simulink model "VcScHv"  (R2023b)
settings: Solver=FixedStepDiscrete  StartTime=0.0  StopTime=1  FixedStep=0.01  RelTol=1e-3
model workspace (MAT data in the model file):
  K_VcScHv_BatteryVoltage_Fallback = Simulink.Parameter
  K_VcScHv_BatteryVoltage_Fallback.Value = 0
  K_VcScHv_BatteryVoltage_Fallback.Description = 'BatteryVoltage Fallback (V)'
  K_VcScHv_BatteryVoltage_Fallback.DataType = 'single'
  K_VcScHv_BatteryVoltage_Fallback.Min = 0
  K_VcScHv_BatteryVoltage_Fallback.Max = 1000
  K_VcScHv_BatteryVoltage_Fallback.Complexity = 'real'
  K_VcScHv_BatteryVoltage_Fallback.Dimensions = [1 1]
  K_VcScHv_BatteryVoltage_Maximum = Simulink.Parameter
  K_VcScHv_BatteryVoltage_Maximum.Value = 10000
  K_VcScHv_BatteryVoltage_Maximum.Description = 'BatteryVoltage Maximum (1)'
  K_VcScHv_BatteryVoltage_Maximum.DataType = 'uint16'
  K_VcScHv_BatteryVoltage_Maximum.Min = 0
  K_VcScHv_BatteryVoltage_Maximum.Max = 10000
  K_VcScHv_BatteryVoltage_Maximum.Complexity = 'real'
  K_VcScHv_BatteryVoltage_Maximum.Dimensions = [1 1]
  K_VcScHv_BatteryVoltage_Minimum = Simulink.Parameter
  K_VcScHv_BatteryVoltage_Minimum.Value = 0
  K_VcScHv_BatteryVoltage_Minimum.Description = 'BatteryVoltage Minimum (1)'
  K_VcScHv_BatteryVoltage_Minimum.DataType = 'uint16'
  K_VcScHv_BatteryVoltage_Minimum.Min = 0
  K_VcScHv_BatteryVoltage_Minimum.Max = 10000
  K_VcScHv_BatteryVoltage_Minimum.Complexity = 'real'
  K_VcScHv_BatteryVoltage_Minimum.Dimensions = [1 1]
  K_VcScHv_BatteryVoltage_Offset = Simulink.Parameter
  K_VcScHv_BatteryVoltage_Offset.Value = 0
  K_VcScHv_BatteryVoltage_Offset.Description = 'BatteryVoltage Offset (V)'
  K_VcScHv_BatteryVoltage_Offset.DataType = 'single'
  K_VcScHv_BatteryVoltage_Offset.Min = 0
  K_VcScHv_BatteryVoltage_Offset.Max = 1000
  K_VcScHv_BatteryVoltage_Offset.Complexity = 'real'
  K_VcScHv_BatteryVoltage_Offset.Dimensions = [1 1]
  K_VcScHv_BatteryVoltage_Scale = Simulink.Parameter
  K_VcScHv_BatteryVoltage_Scale.Value = 0.1
  K_VcScHv_BatteryVoltage_Scale.Description = 'BatteryVoltage Scale (1)'
  K_VcScHv_BatteryVoltage_Scale.DataType = 'single'
  K_VcScHv_BatteryVoltage_Scale.Min = 0
  K_VcScHv_BatteryVoltage_Scale.Max = 100
  K_VcScHv_BatteryVoltage_Scale.Complexity = 'real'
  K_VcScHv_BatteryVoltage_Scale.Dimensions = [1 1]
  K_VcScHv_BatteryVoltage_Timeout = Simulink.Parameter
  K_VcScHv_BatteryVoltage_Timeout.Value = 0.05
  K_VcScHv_BatteryVoltage_Timeout.Description = 'BatteryVoltage Timeout (s)'
  K_VcScHv_BatteryVoltage_Timeout.DataType = 'single'
  K_VcScHv_BatteryVoltage_Timeout.Min = 0
  K_VcScHv_BatteryVoltage_Timeout.Max = 10
  K_VcScHv_BatteryVoltage_Timeout.Complexity = 'real'
  K_VcScHv_BatteryVoltage_Timeout.Dimensions = [1 1]
  K_VcScHv_ChargeEnable_Fallback = Simulink.Parameter
  K_VcScHv_ChargeEnable_Fallback.Value = 0
  K_VcScHv_ChargeEnable_Fallback.Description = 'ChargeEnable Fallback (boolean)'
  K_VcScHv_ChargeEnable_Fallback.DataType = 'boolean'
  K_VcScHv_ChargeEnable_Fallback.Min = 0
  K_VcScHv_ChargeEnable_Fallback.Max = 1
  K_VcScHv_ChargeEnable_Fallback.Complexity = 'real'
  K_VcScHv_ChargeEnable_Fallback.Dimensions = [1 1]
  K_VcScHv_ChargeEnable_Timeout = Simulink.Parameter
  K_VcScHv_ChargeEnable_Timeout.Value = 0.05
  K_VcScHv_ChargeEnable_Timeout.Description = 'ChargeEnable Timeout (s)'
  K_VcScHv_ChargeEnable_Timeout.DataType = 'single'
  K_VcScHv_ChargeEnable_Timeout.Min = 0
  K_VcScHv_ChargeEnable_Timeout.Max = 10
  K_VcScHv_ChargeEnable_Timeout.Complexity = 'real'
  K_VcScHv_ChargeEnable_Timeout.Dimensions = [1 1]
  K_VcScHv_ContactorFeedback_Fallback = Simulink.Parameter
  K_VcScHv_ContactorFeedback_Fallback.Value = 0
  K_VcScHv_ContactorFeedback_Fallback.Description = 'ContactorFeedback Fallback (boolean)'
  K_VcScHv_ContactorFeedback_Fallback.DataType = 'boolean'
  K_VcScHv_ContactorFeedback_Fallback.Min = 0
  K_VcScHv_ContactorFeedback_Fallback.Max = 1
  K_VcScHv_ContactorFeedback_Fallback.Complexity = 'real'
  K_VcScHv_ContactorFeedback_Fallback.Dimensions = [1 1]
  K_VcScHv_ContactorFeedback_Timeout = Simulink.Parameter
  K_VcScHv_ContactorFeedback_Timeout.Value = 0.05
  K_VcScHv_ContactorFeedback_Timeout.Description = 'ContactorFeedback Timeout (s)'
  K_VcScHv_ContactorFeedback_Timeout.DataType = 'single'
  K_VcScHv_ContactorFeedback_Timeout.Min = 0
  K_VcScHv_ContactorFeedback_Timeout.Max = 10
  K_VcScHv_ContactorFeedback_Timeout.Complexity = 'real'
  K_VcScHv_ContactorFeedback_Timeout.Dimensions = [1 1]
  K_VcScHv_CrashSignal_Fallback = Simulink.Parameter
  K_VcScHv_CrashSignal_Fallback.Value = 1
  K_VcScHv_CrashSignal_Fallback.Description = 'CrashSignal Fallback (boolean)'
  K_VcScHv_CrashSignal_Fallback.DataType = 'boolean'
  K_VcScHv_CrashSignal_Fallback.Min = 0
  K_VcScHv_CrashSignal_Fallback.Max = 1
  K_VcScHv_CrashSignal_Fallback.Complexity = 'real'
  K_VcScHv_CrashSignal_Fallback.Dimensions = [1 1]
  K_VcScHv_CrashSignal_Timeout = Simulink.Parameter
  K_VcScHv_CrashSignal_Timeout.Value = 0.05
  K_VcScHv_CrashSignal_Timeout.Description = 'CrashSignal Timeout (s)'
  K_VcScHv_CrashSignal_Timeout.DataType = 'single'
  K_VcScHv_CrashSignal_Timeout.Min = 0
  K_VcScHv_CrashSignal_Timeout.Max = 10
  K_VcScHv_CrashSignal_Timeout.Complexity = 'real'
  K_VcScHv_CrashSignal_Timeout.Dimensions = [1 1]
  K_VcScHv_DcLinkVoltage_Fallback = Simulink.Parameter
  K_VcScHv_DcLinkVoltage_Fallback.Value = 0
  K_VcScHv_DcLinkVoltage_Fallback.Description = 'DcLinkVoltage Fallback (V)'
  K_VcScHv_DcLinkVoltage_Fallback.DataType = 'single'
  K_VcScHv_DcLinkVoltage_Fallback.Min = 0
  K_VcScHv_DcLinkVoltage_Fallback.Max = 1000
  K_VcScHv_DcLinkVoltage_Fallback.Complexity = 'real'
  K_VcScHv_DcLinkVoltage_Fallback.Dimensions = [1 1]
  K_VcScHv_DcLinkVoltage_Maximum = Simulink.Parameter
  K_VcScHv_DcLinkVoltage_Maximum.Value = 10000
  K_VcScHv_DcLinkVoltage_Maximum.Description = 'DcLinkVoltage Maximum (1)'
  K_VcScHv_DcLinkVoltage_Maximum.DataType = 'uint16'
  K_VcScHv_DcLinkVoltage_Maximum.Min = 0
  K_VcScHv_DcLinkVoltage_Maximum.Max = 10000
  K_VcScHv_DcLinkVoltage_Maximum.Complexity = 'real'
  K_VcScHv_DcLinkVoltage_Maximum.Dimensions = [1 1]
  K_VcScHv_DcLinkVoltage_Minimum = Simulink.Parameter
  K_VcScHv_DcLinkVoltage_Minimum.Value = 0
  K_VcScHv_DcLinkVoltage_Minimum.Description = 'DcLinkVoltage Minimum (1)'
  K_VcScHv_DcLinkVoltage_Minimum.DataType = 'uint16'
  K_VcScHv_DcLinkVoltage_Minimum.Min = 0
  K_VcScHv_DcLinkVoltage_Minimum.Max = 10000
  K_VcScHv_DcLinkVoltage_Minimum.Complexity = 'real'
  K_VcScHv_DcLinkVoltage_Minimum.Dimensions = [1 1]
  K_VcScHv_DcLinkVoltage_Offset = Simulink.Parameter
  K_VcScHv_DcLinkVoltage_Offset.Value = 0
  K_VcScHv_DcLinkVoltage_Offset.Description = 'DcLinkVoltage Offset (V)'
  K_VcScHv_DcLinkVoltage_Offset.DataType = 'single'
  K_VcScHv_DcLinkVoltage_Offset.Min = 0
  K_VcScHv_DcLinkVoltage_Offset.Max = 1000
  K_VcScHv_DcLinkVoltage_Offset.Complexity = 'real'
  K_VcScHv_DcLinkVoltage_Offset.Dimensions = [1 1]
  K_VcScHv_DcLinkVoltage_Scale = Simulink.Parameter
  K_VcScHv_DcLinkVoltage_Scale.Value = 0.1
  K_VcScHv_DcLinkVoltage_Scale.Description = 'DcLinkVoltage Scale (1)'
  K_VcScHv_DcLinkVoltage_Scale.DataType = 'single'
  K_VcScHv_DcLinkVoltage_Scale.Min = 0
  K_VcScHv_DcLinkVoltage_Scale.Max = 100
  K_VcScHv_DcLinkVoltage_Scale.Complexity = 'real'
  K_VcScHv_DcLinkVoltage_Scale.Dimensions = [1 1]
  K_VcScHv_DcLinkVoltage_Timeout = Simulink.Parameter
  K_VcScHv_DcLinkVoltage_Timeout.Value = 0.05
  K_VcScHv_DcLinkVoltage_Timeout.Description = 'DcLinkVoltage Timeout (s)'
  K_VcScHv_DcLinkVoltage_Timeout.DataType = 'single'
  K_VcScHv_DcLinkVoltage_Timeout.Min = 0
  K_VcScHv_DcLinkVoltage_Timeout.Max = 10
  K_VcScHv_DcLinkVoltage_Timeout.Complexity = 'real'
  K_VcScHv_DcLinkVoltage_Timeout.Dimensions = [1 1]
  K_VcScHv_DriveEnable_Fallback = Simulink.Parameter
  K_VcScHv_DriveEnable_Fallback.Value = 0
  K_VcScHv_DriveEnable_Fallback.Description = 'DriveEnable Fallback (boolean)'
  K_VcScHv_DriveEnable_Fallback.DataType = 'boolean'
  K_VcScHv_DriveEnable_Fallback.Min = 0
  K_VcScHv_DriveEnable_Fallback.Max = 1
  K_VcScHv_DriveEnable_Fallback.Complexity = 'real'
  K_VcScHv_DriveEnable_Fallback.Dimensions = [1 1]
  K_VcScHv_DriveEnable_Timeout = Simulink.Parameter
  K_VcScHv_DriveEnable_Timeout.Value = 0.05
  K_VcScHv_DriveEnable_Timeout.Description = 'DriveEnable Timeout (s)'
  K_VcScHv_DriveEnable_Timeout.DataType = 'single'
  K_VcScHv_DriveEnable_Timeout.Min = 0
  K_VcScHv_DriveEnable_Timeout.Max = 10
  K_VcScHv_DriveEnable_Timeout.Complexity = 'real'
  K_VcScHv_DriveEnable_Timeout.Dimensions = [1 1]
  K_VcScHv_IsolationResistance_Fallback = Simulink.Parameter
  K_VcScHv_IsolationResistance_Fallback.Value = 0
  K_VcScHv_IsolationResistance_Fallback.Description = 'IsolationResistance Fallback (ohm)'
  K_VcScHv_IsolationResistance_Fallback.DataType = 'single'
  K_VcScHv_IsolationResistance_Fallback.Min = 0
  K_VcScHv_IsolationResistance_Fallback.Max = 2000000
  K_VcScHv_IsolationResistance_Fallback.Complexity = 'real'
  K_VcScHv_IsolationResistance_Fallback.Dimensions = [1 1]
  K_VcScHv_IsolationResistance_Maximum = Simulink.Parameter
  K_VcScHv_IsolationResistance_Maximum.Value = 2000000
  K_VcScHv_IsolationResistance_Maximum.Description = 'IsolationResistance Maximum (ohm)'
  K_VcScHv_IsolationResistance_Maximum.DataType = 'uint32'
  K_VcScHv_IsolationResistance_Maximum.Min = 0
  K_VcScHv_IsolationResistance_Maximum.Max = 2000000
  K_VcScHv_IsolationResistance_Maximum.Complexity = 'real'
  K_VcScHv_IsolationResistance_Maximum.Dimensions = [1 1]
  K_VcScHv_IsolationResistance_Minimum = Simulink.Parameter
  K_VcScHv_IsolationResistance_Minimum.Value = 0
  K_VcScHv_IsolationResistance_Minimum.Description = 'IsolationResistance Minimum (ohm)'
  K_VcScHv_IsolationResistance_Minimum.DataType = 'uint32'
  K_VcScHv_IsolationResistance_Minimum.Min = 0
  K_VcScHv_IsolationResistance_Minimum.Max = 2000000
  K_VcScHv_IsolationResistance_Minimum.Complexity = 'real'
  K_VcScHv_IsolationResistance_Minimum.Dimensions = [1 1]
  K_VcScHv_IsolationResistance_Offset = Simulink.Parameter
  K_VcScHv_IsolationResistance_Offset.Value = 0
  K_VcScHv_IsolationResistance_Offset.Description = 'IsolationResistance Offset (ohm)'
  K_VcScHv_IsolationResistance_Offset.DataType = 'single'
  K_VcScHv_IsolationResistance_Offset.Min = 0
  K_VcScHv_IsolationResistance_Offset.Max = 2000000
  K_VcScHv_IsolationResistance_Offset.Complexity = 'real'
  K_VcScHv_IsolationResistance_Offset.Dimensions = [1 1]
  K_VcScHv_IsolationResistance_Scale = Simulink.Parameter
  K_VcScHv_IsolationResistance_Scale.Value = 1
  K_VcScHv_IsolationResistance_Scale.Description = 'IsolationResistance Scale (1)'
  K_VcScHv_IsolationResistance_Scale.DataType = 'single'
  K_VcScHv_IsolationResistance_Scale.Min = 0
  K_VcScHv_IsolationResistance_Scale.Max = 100
  K_VcScHv_IsolationResistance_Scale.Complexity = 'real'
  K_VcScHv_IsolationResistance_Scale.Dimensions = [1 1]
  K_VcScHv_IsolationResistance_Timeout = Simulink.Parameter
  K_VcScHv_IsolationResistance_Timeout.Value = 0.05
  K_VcScHv_IsolationResistance_Timeout.Description = 'IsolationResistance Timeout (s)'
  K_VcScHv_IsolationResistance_Timeout.DataType = 'single'
  K_VcScHv_IsolationResistance_Timeout.Min = 0
  K_VcScHv_IsolationResistance_Timeout.Max = 10
  K_VcScHv_IsolationResistance_Timeout.Complexity = 'real'
  K_VcScHv_IsolationResistance_Timeout.Dimensions = [1 1]
  K_VcScHv_PrechargeFeedback_Fallback = Simulink.Parameter
  K_VcScHv_PrechargeFeedback_Fallback.Value = 0
  K_VcScHv_PrechargeFeedback_Fallback.Description = 'PrechargeFeedback Fallback (boolean)'
  K_VcScHv_PrechargeFeedback_Fallback.DataType = 'boolean'
  K_VcScHv_PrechargeFeedback_Fallback.Min = 0
  K_VcScHv_PrechargeFeedback_Fallback.Max = 1
  K_VcScHv_PrechargeFeedback_Fallback.Complexity = 'real'
  K_VcScHv_PrechargeFeedback_Fallback.Dimensions = [1 1]
  K_VcScHv_PrechargeFeedback_Timeout = Simulink.Parameter
  K_VcScHv_PrechargeFeedback_Timeout.Value = 0.05
  K_VcScHv_PrechargeFeedback_Timeout.Description = 'PrechargeFeedback Timeout (s)'
  K_VcScHv_PrechargeFeedback_Timeout.DataType = 'single'
  K_VcScHv_PrechargeFeedback_Timeout.Min = 0
  K_VcScHv_PrechargeFeedback_Timeout.Max = 10
  K_VcScHv_PrechargeFeedback_Timeout.Complexity = 'real'
  K_VcScHv_PrechargeFeedback_Timeout.Dimensions = [1 1]
libraries: simulink x1
(part 1 of 2)
Description:
  | Synthetic reality proxy: high_voltage_sequence. Local engineering values; not internal production calibration.
settings Model: Creator=曹博弢  LastModifiedBy=曹博弢
settings DataIOCC: SignalLogging=off
settings OptimizationCC: EnhancedBackFolding=on  PassReuseOutputArgsAs=Individual arguments  ZeroExternalMemoryAtStartup=off  ZeroInternalMemoryAtStartup=off  OptimizeBlockOrder=speed  DifferentSizesBufferReuse=on  OptimizationCustomize=off  EfficientTunableParamExpr=on
settings DebuggingCC: ParameterTunabilityLossMsg=error
settings SFSimCC: MATLABDynamicMemAlloc=off
settings RTWCC: Description=Embedded Coder  SystemTargetFile=ert.tlc  GenCodeOnly=on  TemplateMakefile=ert_default_tmf
settings CodeAppCC: ForceParamTrailComments=on  IgnoreCustomStorageClasses=off  OperatorAnnotations=on  SimulinkDataObjDesc=on  SFDataObjDesc=on  InsertBlockDesc=on
settings ERTTargetCC: TargetLangStandard=C99 (ISO)  GenerateSampleERTMain=on  ERTCustomFileTemplate=example_file_process.tlc

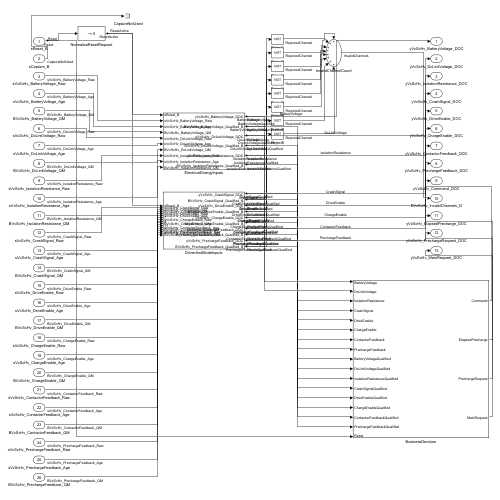
[thumbnail: Simulink's stored preview of the top-level diagram]
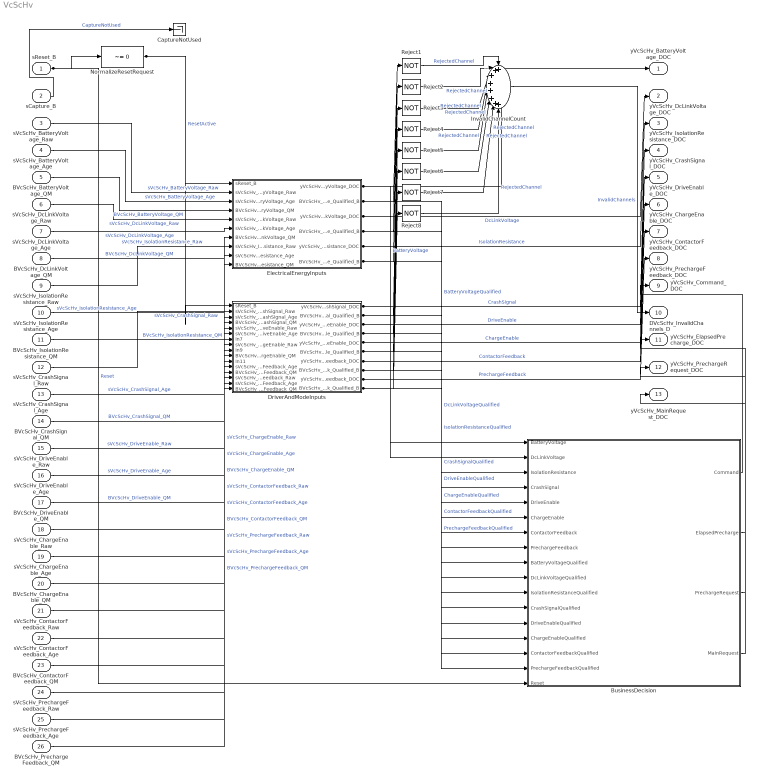
== system VcScHv ==
  sReset_B : Inport  OutDataTypeStr=boolean  Interpolate=off
  sCapture_B : Inport  Port=2  OutDataTypeStr=boolean  Interpolate=off
  sVcScHv_BatteryVoltage_Raw : Inport  Port=3  OutDataTypeStr=uint16  Interpolate=off
  sVcScHv_BatteryVoltage_Age : Inport  Port=4  OutDataTypeStr=single  Interpolate=off
  BVcScHv_BatteryVoltage_QM : Inport  Port=5  OutDataTypeStr=boolean  Interpolate=off
  sVcScHv_DcLinkVoltage_Raw : Inport  Port=6  OutDataTypeStr=uint16  Interpolate=off
  sVcScHv_DcLinkVoltage_Age : Inport  Port=7  OutDataTypeStr=single  Interpolate=off
  BVcScHv_DcLinkVoltage_QM : Inport  Port=8  OutDataTypeStr=boolean  Interpolate=off
  sVcScHv_IsolationResistance_Raw : Inport  Port=9  OutDataTypeStr=uint32  Interpolate=off
  sVcScHv_IsolationResistance_Age : Inport  Port=10  OutDataTypeStr=single  Interpolate=off
  BVcScHv_IsolationResistance_QM : Inport  Port=11  OutDataTypeStr=boolean  Interpolate=off
  sVcScHv_CrashSignal_Raw : Inport  Port=12  OutDataTypeStr=boolean  Interpolate=off
  sVcScHv_CrashSignal_Age : Inport  Port=13  OutDataTypeStr=single  Interpolate=off
  BVcScHv_CrashSignal_QM : Inport  Port=14  OutDataTypeStr=boolean  Interpolate=off
  sVcScHv_DriveEnable_Raw : Inport  Port=15  OutDataTypeStr=boolean  Interpolate=off
  sVcScHv_DriveEnable_Age : Inport  Port=16  OutDataTypeStr=single  Interpolate=off
  BVcScHv_DriveEnable_QM : Inport  Port=17  OutDataTypeStr=boolean  Interpolate=off
  sVcScHv_ChargeEnable_Raw : Inport  Port=18  OutDataTypeStr=boolean  Interpolate=off
  sVcScHv_ChargeEnable_Age : Inport  Port=19  OutDataTypeStr=single  Interpolate=off
  BVcScHv_ChargeEnable_QM : Inport  Port=20  OutDataTypeStr=boolean  Interpolate=off
  sVcScHv_ContactorFeedback_Raw : Inport  Port=21  OutDataTypeStr=boolean  Interpolate=off
  sVcScHv_ContactorFeedback_Age : Inport  Port=22  OutDataTypeStr=single  Interpolate=off
  BVcScHv_ContactorFeedback_QM : Inport  Port=23  OutDataTypeStr=boolean  Interpolate=off
  sVcScHv_PrechargeFeedback_Raw : Inport  Port=24  OutDataTypeStr=boolean  Interpolate=off
  sVcScHv_PrechargeFeedback_Age : Inport  Port=25  OutDataTypeStr=single  Interpolate=off
  BVcScHv_PrechargeFeedback_QM : Inport  Port=26  OutDataTypeStr=boolean  Interpolate=off
  BusinessDecision : Subsystem
  CaptureNotUsed : Terminator
  DriverAndModeInputs : Subsystem
  ElectricalEnergyInputs : Subsystem
  InvalidChannelCount : Sum  Inputs=++++++++  OutDataTypeStr=uint16
  NormalizeResetRequest : simulink/Logic and Bit Operations/Compare To Zero  relop=~=  OutDataTypeStr=boolean
  Reject{1..8} (8 alike) : Logic  Operator=NOT  AllPortsSameDT=off  OutDataTypeStr=boolean
  yVcScHv_BatteryVoltage_DOC : Outport
  yVcScHv_DcLinkVoltage_DOC : Outport  Port=2
  yVcScHv_IsolationResistance_DOC : Outport  Port=3
  yVcScHv_CrashSignal_DOC : Outport  Port=4
  yVcScHv_DriveEnable_DOC : Outport  Port=5
  yVcScHv_ChargeEnable_DOC : Outport  Port=6
  yVcScHv_ContactorFeedback_DOC : Outport  Port=7
  yVcScHv_PrechargeFeedback_DOC : Outport  Port=8
  yVcScHv_Command_DOC : Outport  Port=9
  DVcScHv_InvalidChannels_D : Outport  Port=10
  yVcScHv_ElapsedPrecharge_DOC : Outport  Port=11
  yVcScHv_PrechargeRequest_DOC : Outport  Port=12
  yVcScHv_MainRequest_DOC : Outport  Port=13
  wires:
  sVcScHv_BatteryVoltage_Raw/1 -> ElectricalEnergyInputs/2(sVcScHv_BatteryVoltage_Raw)  "sVcScHv_BatteryVoltage_Raw"
  sVcScHv_BatteryVoltage_Age/1 -> ElectricalEnergyInputs/3(sVcScHv_BatteryVoltage_Age)  "sVcScHv_BatteryVoltage_Age"
  BVcScHv_BatteryVoltage_QM/1 -> ElectricalEnergyInputs/4(BVcScHv_BatteryVoltage_QM)  "BVcScHv_BatteryVoltage_QM"
  sVcScHv_DcLinkVoltage_Raw/1 -> ElectricalEnergyInputs/5(sVcScHv_DcLinkVoltage_Raw)  "sVcScHv_DcLinkVoltage_Raw"
  sVcScHv_DcLinkVoltage_Age/1 -> ElectricalEnergyInputs/6(sVcScHv_DcLinkVoltage_Age)  "sVcScHv_DcLinkVoltage_Age"
  BVcScHv_DcLinkVoltage_QM/1 -> ElectricalEnergyInputs/7(BVcScHv_DcLinkVoltage_QM)  "BVcScHv_DcLinkVoltage_QM"
  sVcScHv_IsolationResistance_Raw/1 -> ElectricalEnergyInputs/8(sVcScHv_IsolationResistance_Raw)  "sVcScHv_IsolationResistance_Raw"
  sVcScHv_IsolationResistance_Age/1 -> ElectricalEnergyInputs/9(sVcScHv_IsolationResistance_Age)  "sVcScHv_IsolationResistance_Age"
  BVcScHv_IsolationResistance_QM/1 -> ElectricalEnergyInputs/10(BVcScHv_IsolationResistance_QM)  "BVcScHv_IsolationResistance_QM"
  sVcScHv_CrashSignal_Raw/1 -> DriverAndModeInputs/2(sVcScHv_CrashSignal_Raw)  "sVcScHv_CrashSignal_Raw"
  sVcScHv_CrashSignal_Age/1 -> DriverAndModeInputs/3(sVcScHv_CrashSignal_Age)  "sVcScHv_CrashSignal_Age"
  BVcScHv_CrashSignal_QM/1 -> DriverAndModeInputs/4(BVcScHv_CrashSignal_QM)  "BVcScHv_CrashSignal_QM"
  sVcScHv_DriveEnable_Raw/1 -> DriverAndModeInputs/5(sVcScHv_DriveEnable_Raw)  "sVcScHv_DriveEnable_Raw"
  sVcScHv_DriveEnable_Age/1 -> DriverAndModeInputs/6(sVcScHv_DriveEnable_Age)  "sVcScHv_DriveEnable_Age"
  BVcScHv_DriveEnable_QM/1 -> DriverAndModeInputs/7(In7)  "BVcScHv_DriveEnable_QM"
  sVcScHv_ChargeEnable_Raw/1 -> DriverAndModeInputs/8(sVcScHv_ChargeEnable_Raw)  "sVcScHv_ChargeEnable_Raw"
  sVcScHv_ChargeEnable_Age/1 -> DriverAndModeInputs/9(In9)  "sVcScHv_ChargeEnable_Age"
  BVcScHv_ChargeEnable_QM/1 -> DriverAndModeInputs/10(BVcScHv_ChargeEnable_QM)  "BVcScHv_ChargeEnable_QM"
  sVcScHv_ContactorFeedback_Raw/1 -> DriverAndModeInputs/11(In11)  "sVcScHv_ContactorFeedback_Raw"
  sVcScHv_ContactorFeedback_Age/1 -> DriverAndModeInputs/12(sVcScHv_ContactorFeedback_Age)  "sVcScHv_ContactorFeedback_Age"
  BVcScHv_ContactorFeedback_QM/1 -> DriverAndModeInputs/13(BVcScHv_ContactorFeedback_QM)  "BVcScHv_ContactorFeedback_QM"
  sVcScHv_PrechargeFeedback_Raw/1 -> DriverAndModeInputs/14(sVcScHv_PrechargeFeedback_Raw)  "sVcScHv_PrechargeFeedback_Raw"
  sVcScHv_PrechargeFeedback_Age/1 -> DriverAndModeInputs/15(sVcScHv_PrechargeFeedback_Age)  "sVcScHv_PrechargeFeedback_Age"
  BVcScHv_PrechargeFeedback_QM/1 -> DriverAndModeInputs/16(BVcScHv_PrechargeFeedback_QM)  "BVcScHv_PrechargeFeedback_QM"
  ElectricalEnergyInputs/1(yVcScHv_BatteryVoltage_DOC) -> yVcScHv_BatteryVoltage_DOC/1, BusinessDecision/1(BatteryVoltage)  "BatteryVoltage"
  ElectricalEnergyInputs/3(yVcScHv_DcLinkVoltage_DOC) -> yVcScHv_DcLinkVoltage_DOC/1, BusinessDecision/2(DcLinkVoltage)  "DcLinkVoltage"
  ElectricalEnergyInputs/5(yVcScHv_IsolationResistance_DOC) -> yVcScHv_IsolationResistance_DOC/1, BusinessDecision/3(IsolationResistance)  "IsolationResistance"
  DriverAndModeInputs/1(yVcScHv_CrashSignal_DOC) -> yVcScHv_CrashSignal_DOC/1, BusinessDecision/4(CrashSignal)  "CrashSignal"
  DriverAndModeInputs/3(yVcScHv_DriveEnable_DOC) -> yVcScHv_DriveEnable_DOC/1, BusinessDecision/5(DriveEnable)  "DriveEnable"
  DriverAndModeInputs/5(yVcScHv_ChargeEnable_DOC) -> yVcScHv_ChargeEnable_DOC/1, BusinessDecision/6(ChargeEnable)  "ChargeEnable"
  DriverAndModeInputs/7(yVcScHv_ContactorFeedback_DOC) -> yVcScHv_ContactorFeedback_DOC/1, BusinessDecision/7(ContactorFeedback)  "ContactorFeedback"
  DriverAndModeInputs/9(yVcScHv_PrechargeFeedback_DOC) -> yVcScHv_PrechargeFeedback_DOC/1, BusinessDecision/8(PrechargeFeedback)  "PrechargeFeedback"
  ElectricalEnergyInputs/2(BVcScHv_BatteryVoltage_Qualified_B) -> Reject1/1, BusinessDecision/9(BatteryVoltageQualified)  "BatteryVoltageQualified"
  Reject1/1 -> InvalidChannelCount/1  "RejectedChannel"
  ElectricalEnergyInputs/4(BVcScHv_DcLinkVoltage_Qualified_B) -> Reject2/1, BusinessDecision/10(DcLinkVoltageQualified)  "DcLinkVoltageQualified"
  Reject2/1 -> InvalidChannelCount/2  "RejectedChannel"
  ElectricalEnergyInputs/6(BVcScHv_IsolationResistance_Qualified_B) -> Reject3/1, BusinessDecision/11(IsolationResistanceQualified)  "IsolationResistanceQualified"
  Reject3/1 -> InvalidChannelCount/3  "RejectedChannel"
  DriverAndModeInputs/2(BVcScHv_CrashSignal_Qualified_B) -> Reject4/1, BusinessDecision/12(CrashSignalQualified)  "CrashSignalQualified"
  Reject4/1 -> InvalidChannelCount/4  "RejectedChannel"
  DriverAndModeInputs/4(BVcScHv_DriveEnable_Qualified_B) -> Reject5/1, BusinessDecision/13(DriveEnableQualified)  "DriveEnableQualified"
  Reject5/1 -> InvalidChannelCount/5  "RejectedChannel"
  DriverAndModeInputs/6(BVcScHv_ChargeEnable_Qualified_B) -> Reject6/1, BusinessDecision/14(ChargeEnableQualified)  "ChargeEnableQualified"
  Reject6/1 -> InvalidChannelCount/6  "RejectedChannel"
  DriverAndModeInputs/8(BVcScHv_ContactorFeedback_Qualified_B) -> Reject7/1, BusinessDecision/15(ContactorFeedbackQualified)  "ContactorFeedbackQualified"
  Reject7/1 -> InvalidChannelCount/7  "RejectedChannel"
  DriverAndModeInputs/10(BVcScHv_PrechargeFeedback_Qualified_B) -> Reject8/1, BusinessDecision/16(PrechargeFeedbackQualified)  "PrechargeFeedbackQualified"
  Reject8/1 -> InvalidChannelCount/8  "RejectedChannel"
  InvalidChannelCount/1 -> DVcScHv_InvalidChannels_D/1  "InvalidChannels"
  sCapture_B/1 -> CaptureNotUsed/1  "CaptureNotUsed"
  sReset_B/1 -> NormalizeResetRequest/1, BusinessDecision/17(Reset)  "Reset"
  NormalizeResetRequest/1 -> ElectricalEnergyInputs/1(sReset_B), DriverAndModeInputs/1(sReset_B)  "ResetActive"
  BusinessDecision/1(Command) -> yVcScHv_Command_DOC/1
  BusinessDecision/2(ElapsedPrecharge) -> yVcScHv_ElapsedPrecharge_DOC/1
  BusinessDecision/3(PrechargeRequest) -> yVcScHv_PrechargeRequest_DOC/1
  BusinessDecision/4(MainRequest) -> yVcScHv_MainRequest_DOC/1

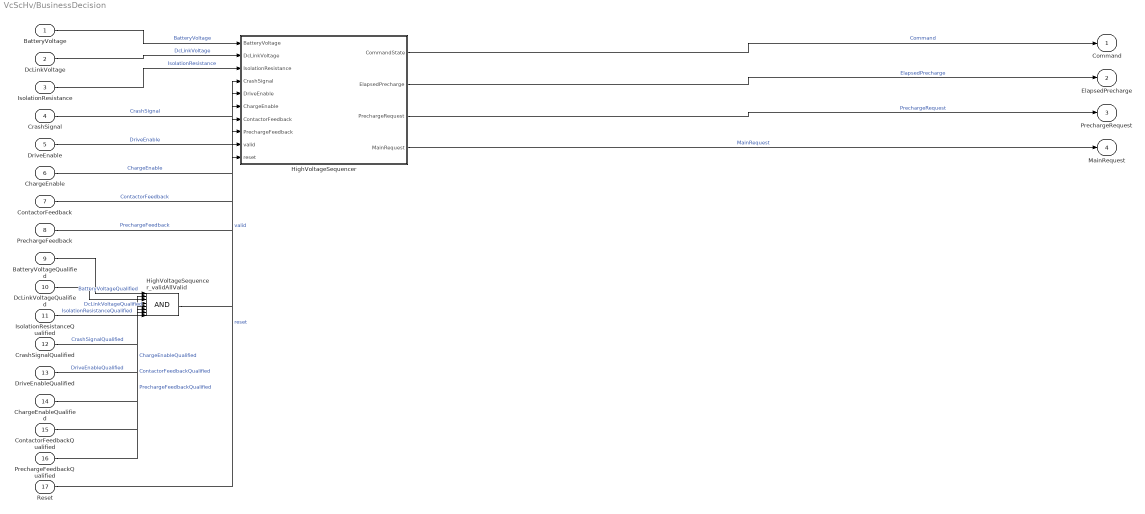
== system VcScHv/BusinessDecision ==
  BatteryVoltage : Inport
  DcLinkVoltage : Inport  Port=2
  IsolationResistance : Inport  Port=3
  CrashSignal : Inport  Port=4
  DriveEnable : Inport  Port=5
  ChargeEnable : Inport  Port=6
  ContactorFeedback : Inport  Port=7
  PrechargeFeedback : Inport  Port=8
  BatteryVoltageQualified : Inport  Port=9
  DcLinkVoltageQualified : Inport  Port=10
  IsolationResistanceQualified : Inport  Port=11
  CrashSignalQualified : Inport  Port=12
  DriveEnableQualified : Inport  Port=13
  ChargeEnableQualified : Inport  Port=14
  ContactorFeedbackQualified : Inport  Port=15
  PrechargeFeedbackQualified : Inport  Port=16
  Reset : Inport  Port=17
  HighVoltageSequencer : Subsystem  Description=Executable responsibility: HighVoltageSequencer. Port units and scenarios are in BusinessBehavior.md and the interface workbook.
  HighVoltageSequencer_validAllValid : Logic  Inputs=8  AllPortsSameDT=off  OutDataTypeStr=boolean
  Command : Outport
  ElapsedPrecharge : Outport  Port=2
  PrechargeRequest : Outport  Port=3
  MainRequest : Outport  Port=4
  wires:
  BatteryVoltage/1 -> HighVoltageSequencer/1(BatteryVoltage)  "BatteryVoltage"
  DcLinkVoltage/1 -> HighVoltageSequencer/2(DcLinkVoltage)  "DcLinkVoltage"
  IsolationResistance/1 -> HighVoltageSequencer/3(IsolationResistance)  "IsolationResistance"
  CrashSignal/1 -> HighVoltageSequencer/4(CrashSignal)  "CrashSignal"
  DriveEnable/1 -> HighVoltageSequencer/5(DriveEnable)  "DriveEnable"
  ChargeEnable/1 -> HighVoltageSequencer/6(ChargeEnable)  "ChargeEnable"
  ContactorFeedback/1 -> HighVoltageSequencer/7(ContactorFeedback)  "ContactorFeedback"
  PrechargeFeedback/1 -> HighVoltageSequencer/8(PrechargeFeedback)  "PrechargeFeedback"
  BatteryVoltageQualified/1 -> HighVoltageSequencer_validAllValid/1  "BatteryVoltageQualified"
  DcLinkVoltageQualified/1 -> HighVoltageSequencer_validAllValid/2  "DcLinkVoltageQualified"
  IsolationResistanceQualified/1 -> HighVoltageSequencer_validAllValid/3  "IsolationResistanceQualified"
  CrashSignalQualified/1 -> HighVoltageSequencer_validAllValid/4  "CrashSignalQualified"
  DriveEnableQualified/1 -> HighVoltageSequencer_validAllValid/5  "DriveEnableQualified"
  ChargeEnableQualified/1 -> HighVoltageSequencer_validAllValid/6  "ChargeEnableQualified"
  ContactorFeedbackQualified/1 -> HighVoltageSequencer_validAllValid/7  "ContactorFeedbackQualified"
  PrechargeFeedbackQualified/1 -> HighVoltageSequencer_validAllValid/8  "PrechargeFeedbackQualified"
  HighVoltageSequencer_validAllValid/1 -> HighVoltageSequencer/9(valid)  "valid"
  Reset/1 -> HighVoltageSequencer/10(reset)  "reset"
  HighVoltageSequencer/1(CommandState) -> Command/1  "Command"
  HighVoltageSequencer/2(ElapsedPrecharge) -> ElapsedPrecharge/1  "ElapsedPrecharge"
  HighVoltageSequencer/3(PrechargeRequest) -> PrechargeRequest/1  "PrechargeRequest"
  HighVoltageSequencer/4(MainRequest) -> MainRequest/1  "MainRequest"

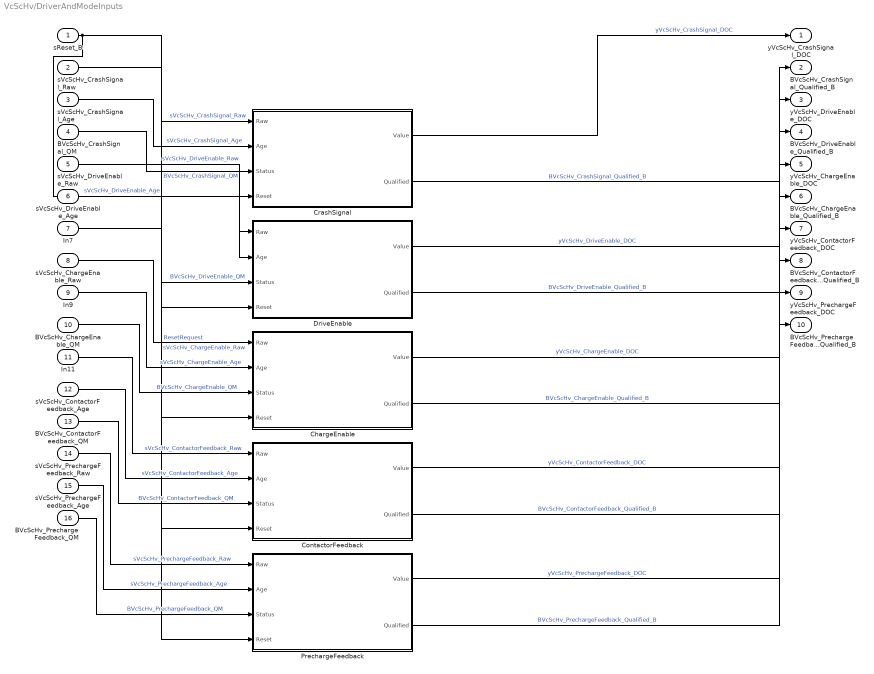
== system VcScHv/DriverAndModeInputs ==
  sReset_B : Inport
  sVcScHv_CrashSignal_Raw : Inport  Port=2
  sVcScHv_CrashSignal_Age : Inport  Port=3
  BVcScHv_CrashSignal_QM : Inport  Port=4
  sVcScHv_DriveEnable_Raw : Inport  Port=5
  sVcScHv_DriveEnable_Age : Inport  Port=6
  In7 : Inport  Port=7
  sVcScHv_ChargeEnable_Raw : Inport  Port=8
  In9 : Inport  Port=9
  BVcScHv_ChargeEnable_QM : Inport  Port=10
  In11 : Inport  Port=11
  sVcScHv_ContactorFeedback_Age : Inport  Port=12
  BVcScHv_ContactorFeedback_QM : Inport  Port=13
  sVcScHv_PrechargeFeedback_Raw : Inport  Port=14
  sVcScHv_PrechargeFeedback_Age : Inport  Port=15
  BVcScHv_PrechargeFeedback_QM : Inport  Port=16
  ChargeEnable : Subsystem  Description=ChargeEnable: digital qualification; raw=boolean, physical=boolean, physical=raw*1+0 boolean  mask{ChannelTimeout=K_VcScHv_ChargeEnable_Timeout}
      mask prompts: ChannelTimeout "Timeout"
      mask help: ChargeEnable: digital qualification; raw=boolean, physical=boolean, physical=raw*1+0 boolean
  ContactorFeedback : Subsystem  Description=ContactorFeedback: digital qualification; raw=boolean, physical=boolean, physical=raw*1+0 boolean  mask{ChannelTimeout=K_VcScHv_ContactorFeedback_Timeout}
      mask prompts: ChannelTimeout "Timeout"
      mask help: ContactorFeedback: digital qualification; raw=boolean, physical=boolean, physical=raw*1+0 boolean
  CrashSignal : Subsystem  Description=CrashSignal: digital qualification; raw=boolean, physical=boolean, physical=raw*1+0 boolean  mask{ChannelTimeout=K_VcScHv_CrashSignal_Timeout}
      mask prompts: ChannelTimeout "Timeout"
      mask help: CrashSignal: digital qualification; raw=boolean, physical=boolean, physical=raw*1+0 boolean
  DriveEnable : Subsystem  Description=DriveEnable: digital qualification; raw=boolean, physical=boolean, physical=raw*1+0 boolean  mask{ChannelTimeout=K_VcScHv_DriveEnable_Timeout}
      mask prompts: ChannelTimeout "Timeout"
      mask help: DriveEnable: digital qualification; raw=boolean, physical=boolean, physical=raw*1+0 boolean
  PrechargeFeedback : Subsystem  Description=PrechargeFeedback: digital qualification; raw=boolean, physical=boolean, physical=raw*1+0 boolean  mask{ChannelTimeout=K_VcScHv_PrechargeFeedback_Timeout}
      mask prompts: ChannelTimeout "Timeout"
      mask help: PrechargeFeedback: digital qualification; raw=boolean, physical=boolean, physical=raw*1+0 boolean
  yVcScHv_CrashSignal_DOC : Outport
  BVcScHv_CrashSignal_Qualified_B : Outport  Port=2
  yVcScHv_DriveEnable_DOC : Outport  Port=3
  BVcScHv_DriveEnable_Qualified_B : Outport  Port=4
  yVcScHv_ChargeEnable_DOC : Outport  Port=5
  BVcScHv_ChargeEnable_Qualified_B : Outport  Port=6
  yVcScHv_ContactorFeedback_DOC : Outport  Port=7
  BVcScHv_ContactorFeedback_Qualified_B : Outport  Port=8
  yVcScHv_PrechargeFeedback_DOC : Outport  Port=9
  BVcScHv_PrechargeFeedback_Qualified_B : Outport  Port=10
  wires:
  sVcScHv_CrashSignal_Raw/1 -> CrashSignal/1(Raw)  "sVcScHv_CrashSignal_Raw"
  sVcScHv_CrashSignal_Age/1 -> CrashSignal/2(Age)  "sVcScHv_CrashSignal_Age"
  BVcScHv_CrashSignal_QM/1 -> CrashSignal/3(Status)  "BVcScHv_CrashSignal_QM"
  sReset_B/1 -> CrashSignal/4(Reset), DriveEnable/4(Reset), ChargeEnable/4(Reset), ContactorFeedback/4(Reset), PrechargeFeedback/4(Reset)  "ResetRequest"
  CrashSignal/1(Value) -> yVcScHv_CrashSignal_DOC/1  "yVcScHv_CrashSignal_DOC"
  CrashSignal/2(Qualified) -> BVcScHv_CrashSignal_Qualified_B/1  "BVcScHv_CrashSignal_Qualified_B"
  sVcScHv_DriveEnable_Raw/1 -> DriveEnable/1(Raw)  "sVcScHv_DriveEnable_Raw"
  sVcScHv_DriveEnable_Age/1 -> DriveEnable/2(Age)  "sVcScHv_DriveEnable_Age"
  In7/1 -> DriveEnable/3(Status)  "BVcScHv_DriveEnable_QM"
  DriveEnable/1(Value) -> yVcScHv_DriveEnable_DOC/1  "yVcScHv_DriveEnable_DOC"
  DriveEnable/2(Qualified) -> BVcScHv_DriveEnable_Qualified_B/1  "BVcScHv_DriveEnable_Qualified_B"
  sVcScHv_ChargeEnable_Raw/1 -> ChargeEnable/1(Raw)  "sVcScHv_ChargeEnable_Raw"
  In9/1 -> ChargeEnable/2(Age)  "sVcScHv_ChargeEnable_Age"
  BVcScHv_ChargeEnable_QM/1 -> ChargeEnable/3(Status)  "BVcScHv_ChargeEnable_QM"
  ChargeEnable/1(Value) -> yVcScHv_ChargeEnable_DOC/1  "yVcScHv_ChargeEnable_DOC"
  ChargeEnable/2(Qualified) -> BVcScHv_ChargeEnable_Qualified_B/1  "BVcScHv_ChargeEnable_Qualified_B"
  In11/1 -> ContactorFeedback/1(Raw)  "sVcScHv_ContactorFeedback_Raw"
  sVcScHv_ContactorFeedback_Age/1 -> ContactorFeedback/2(Age)  "sVcScHv_ContactorFeedback_Age"
  BVcScHv_ContactorFeedback_QM/1 -> ContactorFeedback/3(Status)  "BVcScHv_ContactorFeedback_QM"
  ContactorFeedback/1(Value) -> yVcScHv_ContactorFeedback_DOC/1  "yVcScHv_ContactorFeedback_DOC"
  ContactorFeedback/2(Qualified) -> BVcScHv_ContactorFeedback_Qualified_B/1  "BVcScHv_ContactorFeedback_Qualified_B"
  sVcScHv_PrechargeFeedback_Raw/1 -> PrechargeFeedback/1(Raw)  "sVcScHv_PrechargeFeedback_Raw"
  sVcScHv_PrechargeFeedback_Age/1 -> PrechargeFeedback/2(Age)  "sVcScHv_PrechargeFeedback_Age"
  BVcScHv_PrechargeFeedback_QM/1 -> PrechargeFeedback/3(Status)  "BVcScHv_PrechargeFeedback_QM"
  PrechargeFeedback/1(Value) -> yVcScHv_PrechargeFeedback_DOC/1  "yVcScHv_PrechargeFeedback_DOC"
  PrechargeFeedback/2(Qualified) -> BVcScHv_PrechargeFeedback_Qualified_B/1  "BVcScHv_PrechargeFeedback_Qualified_B"

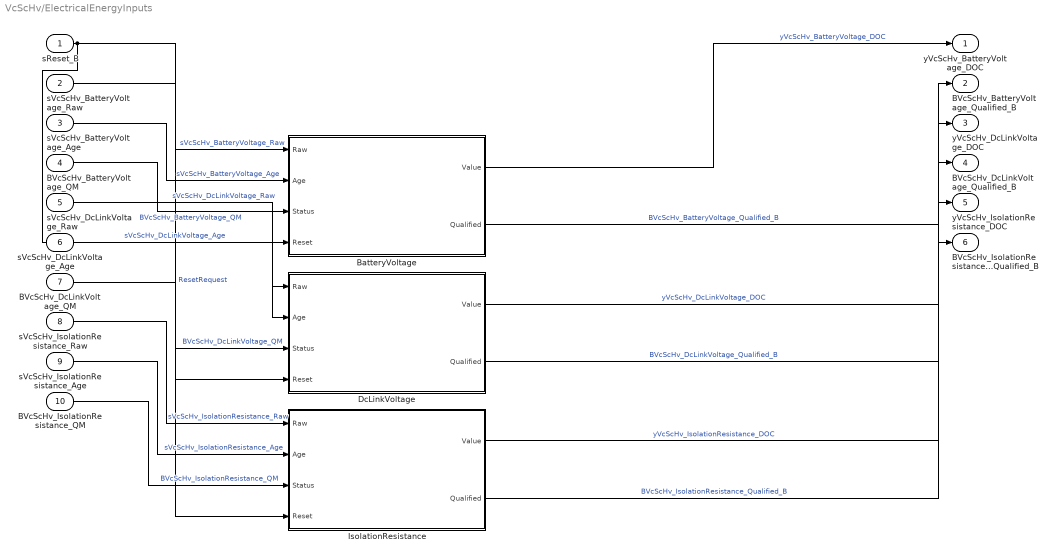
== system VcScHv/ElectricalEnergyInputs ==
  sReset_B : Inport
  sVcScHv_BatteryVoltage_Raw : Inport  Port=2
  sVcScHv_BatteryVoltage_Age : Inport  Port=3
  BVcScHv_BatteryVoltage_QM : Inport  Port=4
  sVcScHv_DcLinkVoltage_Raw : Inport  Port=5
  sVcScHv_DcLinkVoltage_Age : Inport  Port=6
  BVcScHv_DcLinkVoltage_QM : Inport  Port=7
  sVcScHv_IsolationResistance_Raw : Inport  Port=8
  sVcScHv_IsolationResistance_Age : Inport  Port=9
  BVcScHv_IsolationResistance_QM : Inport  Port=10
  BatteryVoltage : Subsystem  Description=BatteryVoltage: analog qualification; raw=uint16, physical=single, physical=raw*0.1+0 V  mask{ChannelMinimum=K_VcScHv_BatteryVoltage_Minimum, ChannelMaximum=K_VcScHv_BatteryVoltage_Maximum, ChannelTimeout=K_VcScHv_BatteryVoltage_Timeout}
      mask prompts: ChannelMinimum "Minimum"; ChannelMaximum "Maximum"; ChannelTimeout "Timeout"
      mask help: BatteryVoltage: analog qualification; raw=uint16, physical=single, physical=raw*0.1+0 V
  DcLinkVoltage : Subsystem  Description=DcLinkVoltage: analog qualification; raw=uint16, physical=single, physical=raw*0.1+0 V  mask{ChannelMinimum=K_VcScHv_DcLinkVoltage_Minimum, ChannelMaximum=K_VcScHv_DcLinkVoltage_Maximum, ChannelTimeout=K_VcScHv_DcLinkVoltage_Timeout}
      mask prompts: ChannelMinimum "Minimum"; ChannelMaximum "Maximum"; ChannelTimeout "Timeout"
      mask help: DcLinkVoltage: analog qualification; raw=uint16, physical=single, physical=raw*0.1+0 V
  IsolationResistance : Subsystem  Description=IsolationResistance: analog qualification; raw=uint32, physical=single, physical=raw*1+0 ohm  mask{ChannelMinimum=K_VcScHv_IsolationResistance_Minimum, ChannelMaximum=K_VcScHv_IsolationResistance_Maximum, ChannelTimeout=K_VcScHv_IsolationResistance_Timeout}
      mask prompts: ChannelMinimum "Minimum"; ChannelMaximum "Maximum"; ChannelTimeout "Timeout"
      mask help: IsolationResistance: analog qualification; raw=uint32, physical=single, physical=raw*1+0 ohm
  yVcScHv_BatteryVoltage_DOC : Outport
  BVcScHv_BatteryVoltage_Qualified_B : Outport  Port=2
  yVcScHv_DcLinkVoltage_DOC : Outport  Port=3
  BVcScHv_DcLinkVoltage_Qualified_B : Outport  Port=4
  yVcScHv_IsolationResistance_DOC : Outport  Port=5
  BVcScHv_IsolationResistance_Qualified_B : Outport  Port=6
  wires:
  sVcScHv_BatteryVoltage_Raw/1 -> BatteryVoltage/1(Raw)  "sVcScHv_BatteryVoltage_Raw"
  sVcScHv_BatteryVoltage_Age/1 -> BatteryVoltage/2(Age)  "sVcScHv_BatteryVoltage_Age"
  BVcScHv_BatteryVoltage_QM/1 -> BatteryVoltage/3(Status)  "BVcScHv_BatteryVoltage_QM"
  sReset_B/1 -> BatteryVoltage/4(Reset), DcLinkVoltage/4(Reset), IsolationResistance/4(Reset)  "ResetRequest"
  BatteryVoltage/1(Value) -> yVcScHv_BatteryVoltage_DOC/1  "yVcScHv_BatteryVoltage_DOC"
  BatteryVoltage/2(Qualified) -> BVcScHv_BatteryVoltage_Qualified_B/1  "BVcScHv_BatteryVoltage_Qualified_B"
  sVcScHv_DcLinkVoltage_Raw/1 -> DcLinkVoltage/1(Raw)  "sVcScHv_DcLinkVoltage_Raw"
  sVcScHv_DcLinkVoltage_Age/1 -> DcLinkVoltage/2(Age)  "sVcScHv_DcLinkVoltage_Age"
  BVcScHv_DcLinkVoltage_QM/1 -> DcLinkVoltage/3(Status)  "BVcScHv_DcLinkVoltage_QM"
  DcLinkVoltage/1(Value) -> yVcScHv_DcLinkVoltage_DOC/1  "yVcScHv_DcLinkVoltage_DOC"
  DcLinkVoltage/2(Qualified) -> BVcScHv_DcLinkVoltage_Qualified_B/1  "BVcScHv_DcLinkVoltage_Qualified_B"
  sVcScHv_IsolationResistance_Raw/1 -> IsolationResistance/1(Raw)  "sVcScHv_IsolationResistance_Raw"
  sVcScHv_IsolationResistance_Age/1 -> IsolationResistance/2(Age)  "sVcScHv_IsolationResistance_Age"
  BVcScHv_IsolationResistance_QM/1 -> IsolationResistance/3(Status)  "BVcScHv_IsolationResistance_QM"
  IsolationResistance/1(Value) -> yVcScHv_IsolationResistance_DOC/1  "yVcScHv_IsolationResistance_DOC"
  IsolationResistance/2(Qualified) -> BVcScHv_IsolationResistance_Qualified_B/1  "BVcScHv_IsolationResistance_Qualified_B"

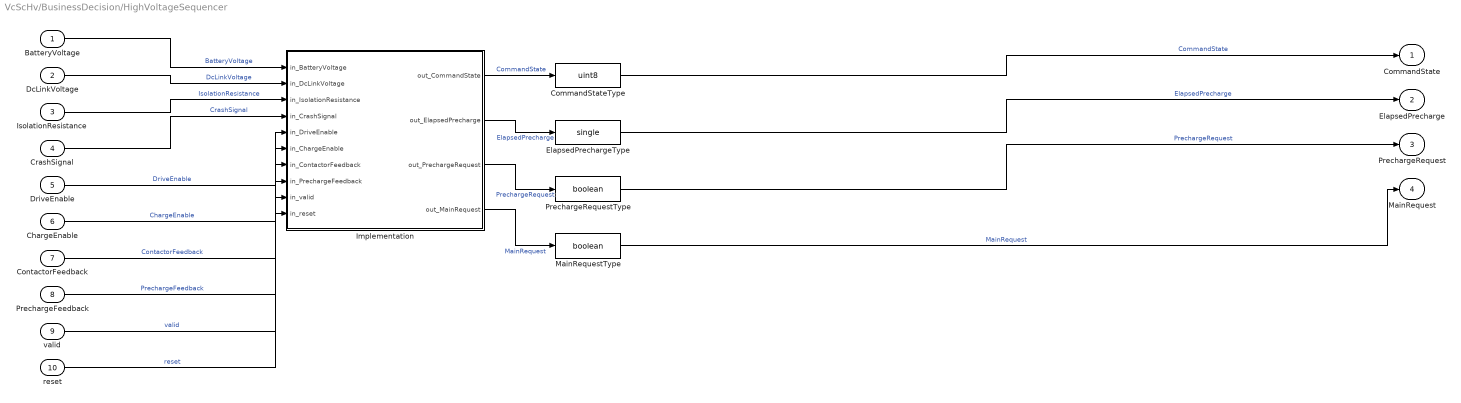
== system VcScHv/BusinessDecision/HighVoltageSequencer ==
  BatteryVoltage : Inport
  DcLinkVoltage : Inport  Port=2
  IsolationResistance : Inport  Port=3
  CrashSignal : Inport  Port=4
  DriveEnable : Inport  Port=5
  ChargeEnable : Inport  Port=6
  ContactorFeedback : Inport  Port=7
  PrechargeFeedback : Inport  Port=8
  valid : Inport  Port=9
  reset : Inport  Port=10
  CommandStateType : DataTypeConversion  OutDataTypeStr=uint8  SaturateOnIntegerOverflow=off  RndMeth=Floor
  ElapsedPrechargeType : DataTypeConversion  OutDataTypeStr=single  SaturateOnIntegerOverflow=off  RndMeth=Floor
  Implementation : MATLAB Function  TreatAsAtomicUnit=on
  MainRequestType : DataTypeConversion  OutDataTypeStr=boolean  SaturateOnIntegerOverflow=off  RndMeth=Floor
  PrechargeRequestType : DataTypeConversion  OutDataTypeStr=boolean  SaturateOnIntegerOverflow=off  RndMeth=Floor
  CommandState : Outport
  ElapsedPrecharge : Outport  Port=2
  PrechargeRequest : Outport  Port=3
  MainRequest : Outport  Port=4
  wires:
  BatteryVoltage/1 -> Implementation/1(in_BatteryVoltage)  "BatteryVoltage"
  DcLinkVoltage/1 -> Implementation/2(in_DcLinkVoltage)  "DcLinkVoltage"
  IsolationResistance/1 -> Implementation/3(in_IsolationResistance)  "IsolationResistance"
  CrashSignal/1 -> Implementation/4(in_CrashSignal)  "CrashSignal"
  DriveEnable/1 -> Implementation/5(in_DriveEnable)  "DriveEnable"
  ChargeEnable/1 -> Implementation/6(in_ChargeEnable)  "ChargeEnable"
  ContactorFeedback/1 -> Implementation/7(in_ContactorFeedback)  "ContactorFeedback"
  PrechargeFeedback/1 -> Implementation/8(in_PrechargeFeedback)  "PrechargeFeedback"
  valid/1 -> Implementation/9(in_valid)  "valid"
  reset/1 -> Implementation/10(in_reset)  "reset"
  Implementation/1(out_CommandState) -> CommandStateType/1  "CommandState"
  CommandStateType/1 -> CommandState/1  "CommandState"
  Implementation/2(out_ElapsedPrecharge) -> ElapsedPrechargeType/1  "ElapsedPrecharge"
  ElapsedPrechargeType/1 -> ElapsedPrecharge/1  "ElapsedPrecharge"
  Implementation/3(out_PrechargeRequest) -> PrechargeRequestType/1  "PrechargeRequest"
  PrechargeRequestType/1 -> PrechargeRequest/1  "PrechargeRequest"
  Implementation/4(out_MainRequest) -> MainRequestType/1  "MainRequest"
  MainRequestType/1 -> MainRequest/1  "MainRequest"

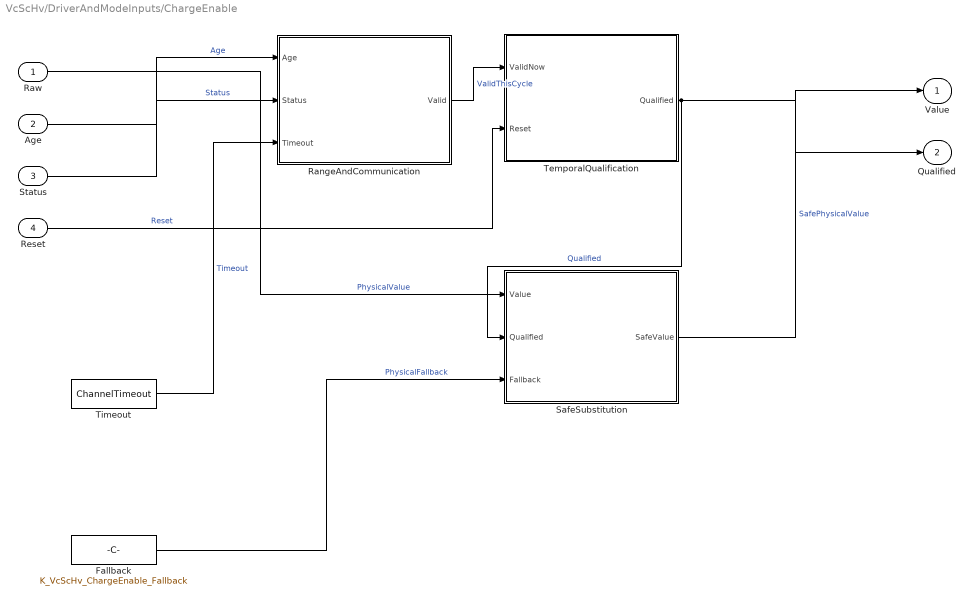
== system VcScHv/DriverAndModeInputs/ChargeEnable ==
  Raw : Inport
  Age : Inport  Port=2
  Status : Inport  Port=3
  Reset : Inport  Port=4
  Fallback : Constant  Value=K_VcScHv_ChargeEnable_Fallback  OutDataTypeStr=boolean
  RangeAndCommunication : Subsystem
  SafeSubstitution : Subsystem
  TemporalQualification : Subsystem
  Timeout : Constant  Value=ChannelTimeout  OutDataTypeStr=single
  Value : Outport
  Qualified : Outport  Port=2
  wires:
  Age/1 -> RangeAndCommunication/1(Age)  "Age"
  Status/1 -> RangeAndCommunication/2(Status)  "Status"
  Timeout/1 -> RangeAndCommunication/3(Timeout)  "Timeout"
  RangeAndCommunication/1(Valid) -> TemporalQualification/1(ValidNow)  "ValidThisCycle"
  Reset/1 -> TemporalQualification/2(Reset)  "Reset"
  Raw/1 -> SafeSubstitution/1(Value)  "PhysicalValue"
  TemporalQualification/1(Qualified) -> SafeSubstitution/2(Qualified), Qualified/1  "Qualified"
  Fallback/1 -> SafeSubstitution/3(Fallback)  "PhysicalFallback"
  SafeSubstitution/1(SafeValue) -> Value/1  "SafePhysicalValue"

== system VcScHv/DriverAndModeInputs/ContactorFeedback ==
  Raw : Inport
  Age : Inport  Port=2
  Status : Inport  Port=3
  Reset : Inport  Port=4
  Fallback : Constant  Value=K_VcScHv_ContactorFeedback_Fallback  OutDataTypeStr=boolean
  RangeAndCommunication : Subsystem
  SafeSubstitution : Subsystem
  TemporalQualification : Subsystem
  Timeout : Constant  Value=ChannelTimeout  OutDataTypeStr=single
  Value : Outport
  Qualified : Outport  Port=2
  wires:
  Age/1 -> RangeAndCommunication/1(Age)  "Age"
  Status/1 -> RangeAndCommunication/2(Status)  "Status"
  Timeout/1 -> RangeAndCommunication/3(Timeout)  "Timeout"
  RangeAndCommunication/1(Valid) -> TemporalQualification/1(ValidNow)  "ValidThisCycle"
  Reset/1 -> TemporalQualification/2(Reset)  "Reset"
  Raw/1 -> SafeSubstitution/1(Value)  "PhysicalValue"
  TemporalQualification/1(Qualified) -> SafeSubstitution/2(Qualified), Qualified/1  "Qualified"
  Fallback/1 -> SafeSubstitution/3(Fallback)  "PhysicalFallback"
  SafeSubstitution/1(SafeValue) -> Value/1  "SafePhysicalValue"

== system VcScHv/DriverAndModeInputs/CrashSignal ==
  Raw : Inport
  Age : Inport  Port=2
  Status : Inport  Port=3
  Reset : Inport  Port=4
  Fallback : Constant  Value=K_VcScHv_CrashSignal_Fallback  OutDataTypeStr=boolean
  RangeAndCommunication : Subsystem
  SafeSubstitution : Subsystem
  TemporalQualification : Subsystem
  Timeout : Constant  Value=ChannelTimeout  OutDataTypeStr=single
  Value : Outport
  Qualified : Outport  Port=2
  wires:
  Age/1 -> RangeAndCommunication/1(Age)  "Age"
  Status/1 -> RangeAndCommunication/2(Status)  "Status"
  Timeout/1 -> RangeAndCommunication/3(Timeout)  "Timeout"
  RangeAndCommunication/1(Valid) -> TemporalQualification/1(ValidNow)  "ValidThisCycle"
  Reset/1 -> TemporalQualification/2(Reset)  "Reset"
  Raw/1 -> SafeSubstitution/1(Value)  "PhysicalValue"
  TemporalQualification/1(Qualified) -> SafeSubstitution/2(Qualified), Qualified/1  "Qualified"
  Fallback/1 -> SafeSubstitution/3(Fallback)  "PhysicalFallback"
  SafeSubstitution/1(SafeValue) -> Value/1  "SafePhysicalValue"

== system VcScHv/DriverAndModeInputs/DriveEnable ==
  Raw : Inport
  Age : Inport  Port=2
  Status : Inport  Port=3
  Reset : Inport  Port=4
  Fallback : Constant  Value=K_VcScHv_DriveEnable_Fallback  OutDataTypeStr=boolean
  RangeAndCommunication : Subsystem
  SafeSubstitution : Subsystem
  TemporalQualification : Subsystem
  Timeout : Constant  Value=ChannelTimeout  OutDataTypeStr=single
  Value : Outport
  Qualified : Outport  Port=2
  wires:
  Age/1 -> RangeAndCommunication/1(Age)  "Age"
  Status/1 -> RangeAndCommunication/2(Status)  "Status"
  Timeout/1 -> RangeAndCommunication/3(Timeout)  "Timeout"
  RangeAndCommunication/1(Valid) -> TemporalQualification/1(ValidNow)  "ValidThisCycle"
  Reset/1 -> TemporalQualification/2(Reset)  "Reset"
  Raw/1 -> SafeSubstitution/1(Value)  "PhysicalValue"
  TemporalQualification/1(Qualified) -> SafeSubstitution/2(Qualified), Qualified/1  "Qualified"
  Fallback/1 -> SafeSubstitution/3(Fallback)  "PhysicalFallback"
  SafeSubstitution/1(SafeValue) -> Value/1  "SafePhysicalValue"

== system VcScHv/DriverAndModeInputs/PrechargeFeedback ==
  Raw : Inport
  Age : Inport  Port=2
  Status : Inport  Port=3
  Reset : Inport  Port=4
  Fallback : Constant  Value=K_VcScHv_PrechargeFeedback_Fallback  OutDataTypeStr=boolean
  RangeAndCommunication : Subsystem
  SafeSubstitution : Subsystem
  TemporalQualification : Subsystem
  Timeout : Constant  Value=ChannelTimeout  OutDataTypeStr=single
  Value : Outport
  Qualified : Outport  Port=2
  wires:
  Age/1 -> RangeAndCommunication/1(Age)  "Age"
  Status/1 -> RangeAndCommunication/2(Status)  "Status"
  Timeout/1 -> RangeAndCommunication/3(Timeout)  "Timeout"
  RangeAndCommunication/1(Valid) -> TemporalQualification/1(ValidNow)  "ValidThisCycle"
  Reset/1 -> TemporalQualification/2(Reset)  "Reset"
  Raw/1 -> SafeSubstitution/1(Value)  "PhysicalValue"
  TemporalQualification/1(Qualified) -> SafeSubstitution/2(Qualified), Qualified/1  "Qualified"
  Fallback/1 -> SafeSubstitution/3(Fallback)  "PhysicalFallback"
  SafeSubstitution/1(SafeValue) -> Value/1  "SafePhysicalValue"

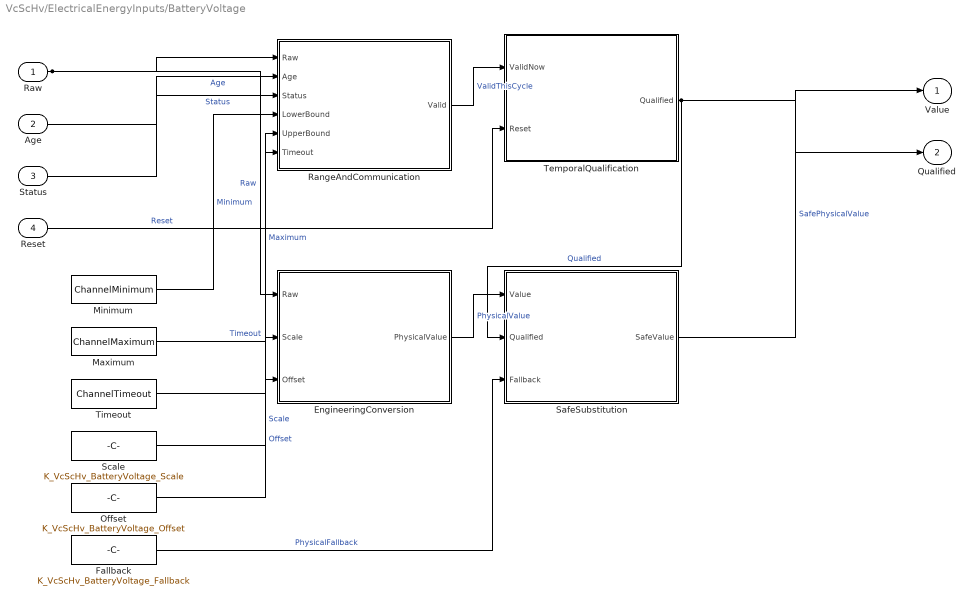
== system VcScHv/ElectricalEnergyInputs/BatteryVoltage ==
  Raw : Inport
  Age : Inport  Port=2
  Status : Inport  Port=3
  Reset : Inport  Port=4
  EngineeringConversion : Subsystem
  Fallback : Constant  Value=K_VcScHv_BatteryVoltage_Fallback  OutDataTypeStr=single
  Maximum : Constant  Value=ChannelMaximum  OutDataTypeStr=uint16
  Minimum : Constant  Value=ChannelMinimum  OutDataTypeStr=uint16
  Offset : Constant  Value=K_VcScHv_BatteryVoltage_Offset  OutDataTypeStr=single
  RangeAndCommunication : Subsystem
  SafeSubstitution : Subsystem
  Scale : Constant  Value=K_VcScHv_BatteryVoltage_Scale  OutDataTypeStr=single
  TemporalQualification : Subsystem
  Timeout : Constant  Value=ChannelTimeout  OutDataTypeStr=single
  Value : Outport
  Qualified : Outport  Port=2
  wires:
  Raw/1 -> RangeAndCommunication/1(Raw), EngineeringConversion/1(Raw)  "Raw"
  Age/1 -> RangeAndCommunication/2(Age)  "Age"
  Status/1 -> RangeAndCommunication/3(Status)  "Status"
  Minimum/1 -> RangeAndCommunication/4(LowerBound)  "Minimum"
  Maximum/1 -> RangeAndCommunication/5(UpperBound)  "Maximum"
  Timeout/1 -> RangeAndCommunication/6(Timeout)  "Timeout"
  RangeAndCommunication/1(Valid) -> TemporalQualification/1(ValidNow)  "ValidThisCycle"
  Reset/1 -> TemporalQualification/2(Reset)  "Reset"
  Scale/1 -> EngineeringConversion/2(Scale)  "Scale"
  Offset/1 -> EngineeringConversion/3(Offset)  "Offset"
  EngineeringConversion/1(PhysicalValue) -> SafeSubstitution/1(Value)  "PhysicalValue"
  TemporalQualification/1(Qualified) -> SafeSubstitution/2(Qualified), Qualified/1  "Qualified"
  Fallback/1 -> SafeSubstitution/3(Fallback)  "PhysicalFallback"
  SafeSubstitution/1(SafeValue) -> Value/1  "SafePhysicalValue"

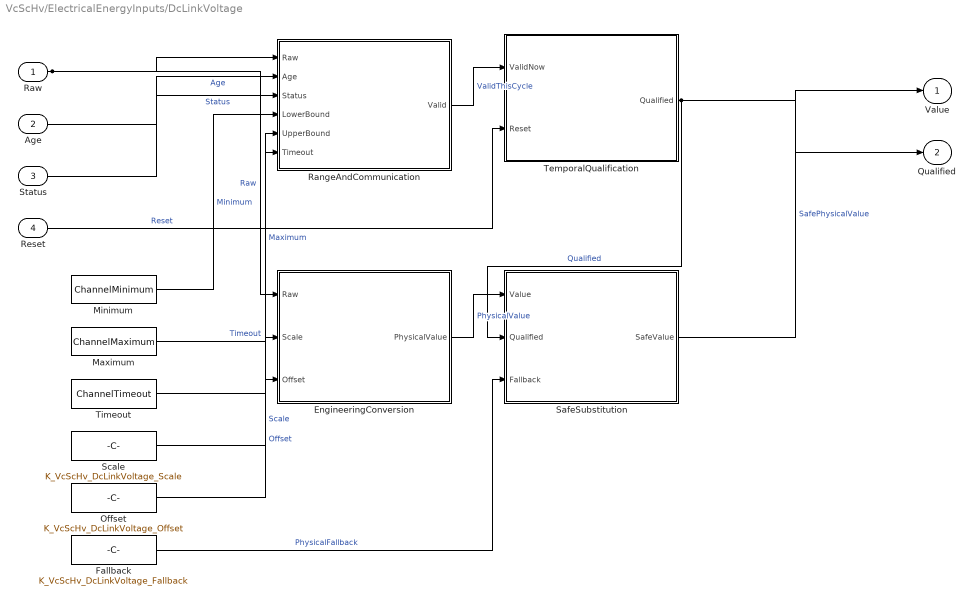
== system VcScHv/ElectricalEnergyInputs/DcLinkVoltage ==
  Raw : Inport
  Age : Inport  Port=2
  Status : Inport  Port=3
  Reset : Inport  Port=4
  EngineeringConversion : Subsystem
  Fallback : Constant  Value=K_VcScHv_DcLinkVoltage_Fallback  OutDataTypeStr=single
  Maximum : Constant  Value=ChannelMaximum  OutDataTypeStr=uint16
  Minimum : Constant  Value=ChannelMinimum  OutDataTypeStr=uint16
  Offset : Constant  Value=K_VcScHv_DcLinkVoltage_Offset  OutDataTypeStr=single
  RangeAndCommunication : Subsystem
  SafeSubstitution : Subsystem
  Scale : Constant  Value=K_VcScHv_DcLinkVoltage_Scale  OutDataTypeStr=single
  TemporalQualification : Subsystem
  Timeout : Constant  Value=ChannelTimeout  OutDataTypeStr=single
  Value : Outport
  Qualified : Outport  Port=2
  wires:
  Raw/1 -> RangeAndCommunication/1(Raw), EngineeringConversion/1(Raw)  "Raw"
  Age/1 -> RangeAndCommunication/2(Age)  "Age"
  Status/1 -> RangeAndCommunication/3(Status)  "Status"
  Minimum/1 -> RangeAndCommunication/4(LowerBound)  "Minimum"
  Maximum/1 -> RangeAndCommunication/5(UpperBound)  "Maximum"
  Timeout/1 -> RangeAndCommunication/6(Timeout)  "Timeout"
  RangeAndCommunication/1(Valid) -> TemporalQualification/1(ValidNow)  "ValidThisCycle"
  Reset/1 -> TemporalQualification/2(Reset)  "Reset"
  Scale/1 -> EngineeringConversion/2(Scale)  "Scale"
  Offset/1 -> EngineeringConversion/3(Offset)  "Offset"
  EngineeringConversion/1(PhysicalValue) -> SafeSubstitution/1(Value)  "PhysicalValue"
  TemporalQualification/1(Qualified) -> SafeSubstitution/2(Qualified), Qualified/1  "Qualified"
  Fallback/1 -> SafeSubstitution/3(Fallback)  "PhysicalFallback"
  SafeSubstitution/1(SafeValue) -> Value/1  "SafePhysicalValue"

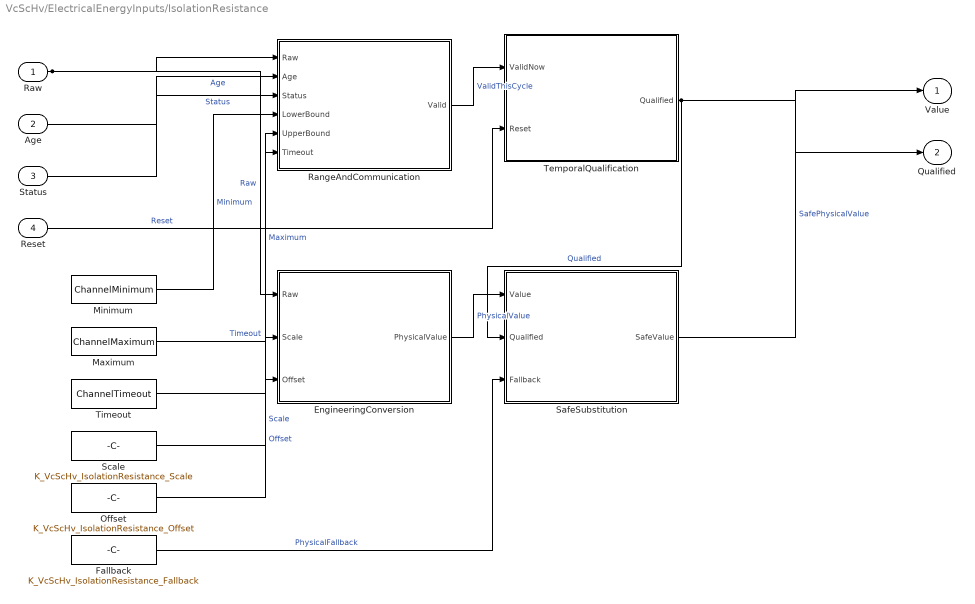
== system VcScHv/ElectricalEnergyInputs/IsolationResistance ==
  Raw : Inport
  Age : Inport  Port=2
  Status : Inport  Port=3
  Reset : Inport  Port=4
  EngineeringConversion : Subsystem
  Fallback : Constant  Value=K_VcScHv_IsolationResistance_Fallback  OutDataTypeStr=single
  Maximum : Constant  Value=ChannelMaximum  OutDataTypeStr=uint32
  Minimum : Constant  Value=ChannelMinimum  OutDataTypeStr=uint32
  Offset : Constant  Value=K_VcScHv_IsolationResistance_Offset  OutDataTypeStr=single
  RangeAndCommunication : Subsystem
  SafeSubstitution : Subsystem
  Scale : Constant  Value=K_VcScHv_IsolationResistance_Scale  OutDataTypeStr=single
  TemporalQualification : Subsystem
  Timeout : Constant  Value=ChannelTimeout  OutDataTypeStr=single
  Value : Outport
  Qualified : Outport  Port=2
  wires:
  Raw/1 -> RangeAndCommunication/1(Raw), EngineeringConversion/1(Raw)  "Raw"
  Age/1 -> RangeAndCommunication/2(Age)  "Age"
  Status/1 -> RangeAndCommunication/3(Status)  "Status"
  Minimum/1 -> RangeAndCommunication/4(LowerBound)  "Minimum"
  Maximum/1 -> RangeAndCommunication/5(UpperBound)  "Maximum"
  Timeout/1 -> RangeAndCommunication/6(Timeout)  "Timeout"
  RangeAndCommunication/1(Valid) -> TemporalQualification/1(ValidNow)  "ValidThisCycle"
  Reset/1 -> TemporalQualification/2(Reset)  "Reset"
  Scale/1 -> EngineeringConversion/2(Scale)  "Scale"
  Offset/1 -> EngineeringConversion/3(Offset)  "Offset"
  EngineeringConversion/1(PhysicalValue) -> SafeSubstitution/1(Value)  "PhysicalValue"
  TemporalQualification/1(Qualified) -> SafeSubstitution/2(Qualified), Qualified/1  "Qualified"
  Fallback/1 -> SafeSubstitution/3(Fallback)  "PhysicalFallback"
  SafeSubstitution/1(SafeValue) -> Value/1  "SafePhysicalValue"

== system VcScHv/DriverAndModeInputs/ChargeEnable/RangeAndCommunication ==
  Age : Inport
  Status : Inport  Port=2
  Timeout : Inport  Port=3
  Fresh : RelationalOperator  Operator=<=  OutDataTypeStr=boolean  RndMeth=Simplest  InputSameDT=off
  NonnegativeAge : RelationalOperator  OutDataTypeStr=boolean  RndMeth=Simplest  InputSameDT=off
  ValidThisCycle : Logic  Inputs=3  AllPortsSameDT=off  OutDataTypeStr=boolean
  ZeroAge : Constant  Value=single(0)
  Valid : Outport
  wires:
  Age/1 -> NonnegativeAge/1, Fresh/1  "Age"
  ZeroAge/1 -> NonnegativeAge/2  "ZeroAge"
  Timeout/1 -> Fresh/2  "Timeout"
  NonnegativeAge/1 -> ValidThisCycle/1  "NonnegativeAge"
  Fresh/1 -> ValidThisCycle/2  "Fresh"
  Status/1 -> ValidThisCycle/3  "Status"
  ValidThisCycle/1 -> Valid/1  "InstantaneousValidity"

== system VcScHv/DriverAndModeInputs/ChargeEnable/SafeSubstitution ==
  Value : Inport
  Qualified : Inport  Port=2
  Fallback : Inport  Port=3
  SelectSafeValue : Switch  Criteria=u2 ~= 0  SaturateOnIntegerOverflow=off  InputSameDT=off
  SafeValue : Outport
  wires:
  Value/1 -> SelectSafeValue/1  "Value"
  Qualified/1 -> SelectSafeValue/2  "Qualified"
  Fallback/1 -> SelectSafeValue/3  "Fallback"
  SelectSafeValue/1 -> SafeValue/1  "SafeValue"

== system VcScHv/DriverAndModeInputs/ChargeEnable/TemporalQualification ==
  ValidNow : Inport
  Reset : Inport  Port=2
  HistoryInput : Logic  AllPortsSameDT=off  OutDataTypeStr=boolean
  PreviousValid : UnitDelay  InitialCondition=false  SampleTime=-1  HasFrameUpgradeWarning=on
  ResetInactive : Logic  Operator=NOT  AllPortsSameDT=off  OutDataTypeStr=boolean
  TwoConsecutiveValid : Logic  Inputs=3  AllPortsSameDT=off  OutDataTypeStr=boolean
  Qualified : Outport
  wires:
  Reset/1 -> ResetInactive/1  "Reset"
  ValidNow/1 -> HistoryInput/1, TwoConsecutiveValid/1  "TwoConsecutiveValid"
  ResetInactive/1 -> HistoryInput/2, TwoConsecutiveValid/3  "TwoConsecutiveValid"
  HistoryInput/1 -> PreviousValid/1  "ValidityHistory"
  PreviousValid/1 -> TwoConsecutiveValid/2  "TwoConsecutiveValid"
  TwoConsecutiveValid/1 -> Qualified/1  "Qualified"

== system VcScHv/DriverAndModeInputs/ContactorFeedback/RangeAndCommunication ==
  Age : Inport
  Status : Inport  Port=2
  Timeout : Inport  Port=3
  Fresh : RelationalOperator  Operator=<=  OutDataTypeStr=boolean  RndMeth=Simplest  InputSameDT=off
  NonnegativeAge : RelationalOperator  OutDataTypeStr=boolean  RndMeth=Simplest  InputSameDT=off
  ValidThisCycle : Logic  Inputs=3  AllPortsSameDT=off  OutDataTypeStr=boolean
  ZeroAge : Constant  Value=single(0)
  Valid : Outport
  wires:
  Age/1 -> NonnegativeAge/1, Fresh/1  "Age"
  ZeroAge/1 -> NonnegativeAge/2  "ZeroAge"
  Timeout/1 -> Fresh/2  "Timeout"
  NonnegativeAge/1 -> ValidThisCycle/1  "NonnegativeAge"
  Fresh/1 -> ValidThisCycle/2  "Fresh"
  Status/1 -> ValidThisCycle/3  "Status"
  ValidThisCycle/1 -> Valid/1  "InstantaneousValidity"

== system VcScHv/DriverAndModeInputs/ContactorFeedback/SafeSubstitution ==
  Value : Inport
  Qualified : Inport  Port=2
  Fallback : Inport  Port=3
  SelectSafeValue : Switch  Criteria=u2 ~= 0  SaturateOnIntegerOverflow=off  InputSameDT=off
  SafeValue : Outport
  wires:
  Value/1 -> SelectSafeValue/1  "Value"
  Qualified/1 -> SelectSafeValue/2  "Qualified"
  Fallback/1 -> SelectSafeValue/3  "Fallback"
  SelectSafeValue/1 -> SafeValue/1  "SafeValue"

== system VcScHv/DriverAndModeInputs/ContactorFeedback/TemporalQualification ==
  ValidNow : Inport
  Reset : Inport  Port=2
  HistoryInput : Logic  AllPortsSameDT=off  OutDataTypeStr=boolean
  PreviousValid : UnitDelay  InitialCondition=false  SampleTime=-1  HasFrameUpgradeWarning=on
  ResetInactive : Logic  Operator=NOT  AllPortsSameDT=off  OutDataTypeStr=boolean
  TwoConsecutiveValid : Logic  Inputs=3  AllPortsSameDT=off  OutDataTypeStr=boolean
  Qualified : Outport
  wires:
  Reset/1 -> ResetInactive/1  "Reset"
  ValidNow/1 -> HistoryInput/1, TwoConsecutiveValid/1  "TwoConsecutiveValid"
  ResetInactive/1 -> HistoryInput/2, TwoConsecutiveValid/3  "TwoConsecutiveValid"
  HistoryInput/1 -> PreviousValid/1  "ValidityHistory"
  PreviousValid/1 -> TwoConsecutiveValid/2  "TwoConsecutiveValid"
  TwoConsecutiveValid/1 -> Qualified/1  "Qualified"

== system VcScHv/DriverAndModeInputs/CrashSignal/RangeAndCommunication ==
  Age : Inport
  Status : Inport  Port=2
  Timeout : Inport  Port=3
  Fresh : RelationalOperator  Operator=<=  OutDataTypeStr=boolean  RndMeth=Simplest  InputSameDT=off
  NonnegativeAge : RelationalOperator  OutDataTypeStr=boolean  RndMeth=Simplest  InputSameDT=off
  ValidThisCycle : Logic  Inputs=3  AllPortsSameDT=off  OutDataTypeStr=boolean
  ZeroAge : Constant  Value=single(0)
  Valid : Outport
  wires:
  Age/1 -> NonnegativeAge/1, Fresh/1  "Age"
  ZeroAge/1 -> NonnegativeAge/2  "ZeroAge"
  Timeout/1 -> Fresh/2  "Timeout"
  NonnegativeAge/1 -> ValidThisCycle/1  "NonnegativeAge"
  Fresh/1 -> ValidThisCycle/2  "Fresh"
  Status/1 -> ValidThisCycle/3  "Status"
  ValidThisCycle/1 -> Valid/1  "InstantaneousValidity"

== system VcScHv/DriverAndModeInputs/CrashSignal/SafeSubstitution ==
  Value : Inport
  Qualified : Inport  Port=2
  Fallback : Inport  Port=3
  SelectSafeValue : Switch  Criteria=u2 ~= 0  SaturateOnIntegerOverflow=off  InputSameDT=off
  SafeValue : Outport
  wires:
  Value/1 -> SelectSafeValue/1  "Value"
  Qualified/1 -> SelectSafeValue/2  "Qualified"
  Fallback/1 -> SelectSafeValue/3  "Fallback"
  SelectSafeValue/1 -> SafeValue/1  "SafeValue"

== system VcScHv/DriverAndModeInputs/CrashSignal/TemporalQualification ==
  ValidNow : Inport
  Reset : Inport  Port=2
  HistoryInput : Logic  AllPortsSameDT=off  OutDataTypeStr=boolean
  PreviousValid : UnitDelay  InitialCondition=false  SampleTime=-1  HasFrameUpgradeWarning=on
  ResetInactive : Logic  Operator=NOT  AllPortsSameDT=off  OutDataTypeStr=boolean
  TwoConsecutiveValid : Logic  Inputs=3  AllPortsSameDT=off  OutDataTypeStr=boolean
  Qualified : Outport
  wires:
  Reset/1 -> ResetInactive/1  "Reset"
  ValidNow/1 -> HistoryInput/1, TwoConsecutiveValid/1  "TwoConsecutiveValid"
  ResetInactive/1 -> HistoryInput/2, TwoConsecutiveValid/3  "TwoConsecutiveValid"
  HistoryInput/1 -> PreviousValid/1  "ValidityHistory"
  PreviousValid/1 -> TwoConsecutiveValid/2  "TwoConsecutiveValid"
  TwoConsecutiveValid/1 -> Qualified/1  "Qualified"

== system VcScHv/DriverAndModeInputs/DriveEnable/RangeAndCommunication ==
  Age : Inport
  Status : Inport  Port=2
  Timeout : Inport  Port=3
  Fresh : RelationalOperator  Operator=<=  OutDataTypeStr=boolean  RndMeth=Simplest  InputSameDT=off
  NonnegativeAge : RelationalOperator  OutDataTypeStr=boolean  RndMeth=Simplest  InputSameDT=off
  ValidThisCycle : Logic  Inputs=3  AllPortsSameDT=off  OutDataTypeStr=boolean
  ZeroAge : Constant  Value=single(0)
  Valid : Outport
  wires:
  Age/1 -> NonnegativeAge/1, Fresh/1  "Age"
  ZeroAge/1 -> NonnegativeAge/2  "ZeroAge"
  Timeout/1 -> Fresh/2  "Timeout"
  NonnegativeAge/1 -> ValidThisCycle/1  "NonnegativeAge"
  Fresh/1 -> ValidThisCycle/2  "Fresh"
  Status/1 -> ValidThisCycle/3  "Status"
  ValidThisCycle/1 -> Valid/1  "InstantaneousValidity"

== system VcScHv/DriverAndModeInputs/DriveEnable/SafeSubstitution ==
  Value : Inport
  Qualified : Inport  Port=2
  Fallback : Inport  Port=3
  SelectSafeValue : Switch  Criteria=u2 ~= 0  SaturateOnIntegerOverflow=off  InputSameDT=off
  SafeValue : Outport
  wires:
  Value/1 -> SelectSafeValue/1  "Value"
  Qualified/1 -> SelectSafeValue/2  "Qualified"
  Fallback/1 -> SelectSafeValue/3  "Fallback"
  SelectSafeValue/1 -> SafeValue/1  "SafeValue"

== system VcScHv/DriverAndModeInputs/DriveEnable/TemporalQualification ==
  ValidNow : Inport
  Reset : Inport  Port=2
  HistoryInput : Logic  AllPortsSameDT=off  OutDataTypeStr=boolean
  PreviousValid : UnitDelay  InitialCondition=false  SampleTime=-1  HasFrameUpgradeWarning=on
  ResetInactive : Logic  Operator=NOT  AllPortsSameDT=off  OutDataTypeStr=boolean
  TwoConsecutiveValid : Logic  Inputs=3  AllPortsSameDT=off  OutDataTypeStr=boolean
  Qualified : Outport
  wires:
  Reset/1 -> ResetInactive/1  "Reset"
  ValidNow/1 -> HistoryInput/1, TwoConsecutiveValid/1  "TwoConsecutiveValid"
  ResetInactive/1 -> HistoryInput/2, TwoConsecutiveValid/3  "TwoConsecutiveValid"
  HistoryInput/1 -> PreviousValid/1  "ValidityHistory"
  PreviousValid/1 -> TwoConsecutiveValid/2  "TwoConsecutiveValid"
  TwoConsecutiveValid/1 -> Qualified/1  "Qualified"

== system VcScHv/DriverAndModeInputs/PrechargeFeedback/RangeAndCommunication ==
  Age : Inport
  Status : Inport  Port=2
  Timeout : Inport  Port=3
  Fresh : RelationalOperator  Operator=<=  OutDataTypeStr=boolean  RndMeth=Simplest  InputSameDT=off
  NonnegativeAge : RelationalOperator  OutDataTypeStr=boolean  RndMeth=Simplest  InputSameDT=off
  ValidThisCycle : Logic  Inputs=3  AllPortsSameDT=off  OutDataTypeStr=boolean
  ZeroAge : Constant  Value=single(0)
  Valid : Outport
  wires:
  Age/1 -> NonnegativeAge/1, Fresh/1  "Age"
  ZeroAge/1 -> NonnegativeAge/2  "ZeroAge"
  Timeout/1 -> Fresh/2  "Timeout"
  NonnegativeAge/1 -> ValidThisCycle/1  "NonnegativeAge"
  Fresh/1 -> ValidThisCycle/2  "Fresh"
  Status/1 -> ValidThisCycle/3  "Status"
  ValidThisCycle/1 -> Valid/1  "InstantaneousValidity"

== system VcScHv/DriverAndModeInputs/PrechargeFeedback/SafeSubstitution ==
  Value : Inport
  Qualified : Inport  Port=2
  Fallback : Inport  Port=3
  SelectSafeValue : Switch  Criteria=u2 ~= 0  SaturateOnIntegerOverflow=off  InputSameDT=off
  SafeValue : Outport
  wires:
  Value/1 -> SelectSafeValue/1  "Value"
  Qualified/1 -> SelectSafeValue/2  "Qualified"
  Fallback/1 -> SelectSafeValue/3  "Fallback"
  SelectSafeValue/1 -> SafeValue/1  "SafeValue"

== system VcScHv/DriverAndModeInputs/PrechargeFeedback/TemporalQualification ==
  ValidNow : Inport
  Reset : Inport  Port=2
  HistoryInput : Logic  AllPortsSameDT=off  OutDataTypeStr=boolean
  PreviousValid : UnitDelay  InitialCondition=false  SampleTime=-1  HasFrameUpgradeWarning=on
  ResetInactive : Logic  Operator=NOT  AllPortsSameDT=off  OutDataTypeStr=boolean
  TwoConsecutiveValid : Logic  Inputs=3  AllPortsSameDT=off  OutDataTypeStr=boolean
  Qualified : Outport
  wires:
  Reset/1 -> ResetInactive/1  "Reset"
  ValidNow/1 -> HistoryInput/1, TwoConsecutiveValid/1  "TwoConsecutiveValid"
  ResetInactive/1 -> HistoryInput/2, TwoConsecutiveValid/3  "TwoConsecutiveValid"
  HistoryInput/1 -> PreviousValid/1  "ValidityHistory"
  PreviousValid/1 -> TwoConsecutiveValid/2  "TwoConsecutiveValid"
  TwoConsecutiveValid/1 -> Qualified/1  "Qualified"

== system VcScHv/ElectricalEnergyInputs/BatteryVoltage/EngineeringConversion ==
  Raw : Inport
  Scale : Inport  Port=2
  Offset : Inport  Port=3
  ApplyOffset : Sum
  RawToPhysicalArithmetic : DataTypeConversion  OutDataTypeStr=single  SaturateOnIntegerOverflow=off  RndMeth=Floor
  ScaleRaw : Product
  PhysicalValue : Outport
  wires:
  Raw/1 -> RawToPhysicalArithmetic/1  "TypedRaw"
  RawToPhysicalArithmetic/1 -> ScaleRaw/1  "RawAsSingle"
  Scale/1 -> ScaleRaw/2  "Scale"
  ScaleRaw/1 -> ApplyOffset/1  "Scaled"
  Offset/1 -> ApplyOffset/2  "Offset"
  ApplyOffset/1 -> PhysicalValue/1  "PhysicalValue"
